simulink model "Lab2"  (R2022a)
settings: Solver=VariableStepAuto  StartTime=0.0  StopTime=100  RelTol=1e-3
values from neighbouring files (symbols this model uses):
  a = 1    [code2.m]
  am = 2    [code2.m]
  b = 0.5    [code2.m]
  bm = 2    [code2.m]
  gamma_tild = gamma*b/am    (= 5)    [code2.m]
settings Model: Creator=fades  LastModifiedBy=fades

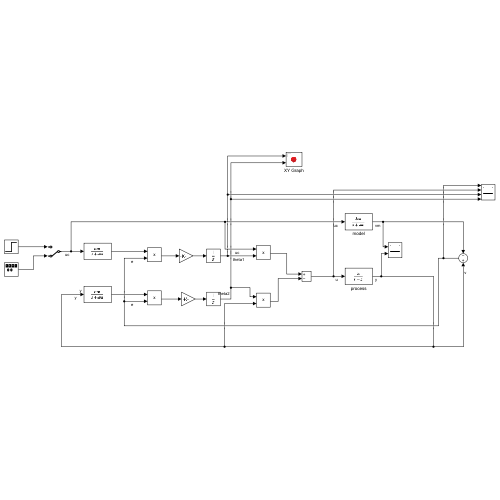
[thumbnail: Simulink's stored preview of the top-level diagram]
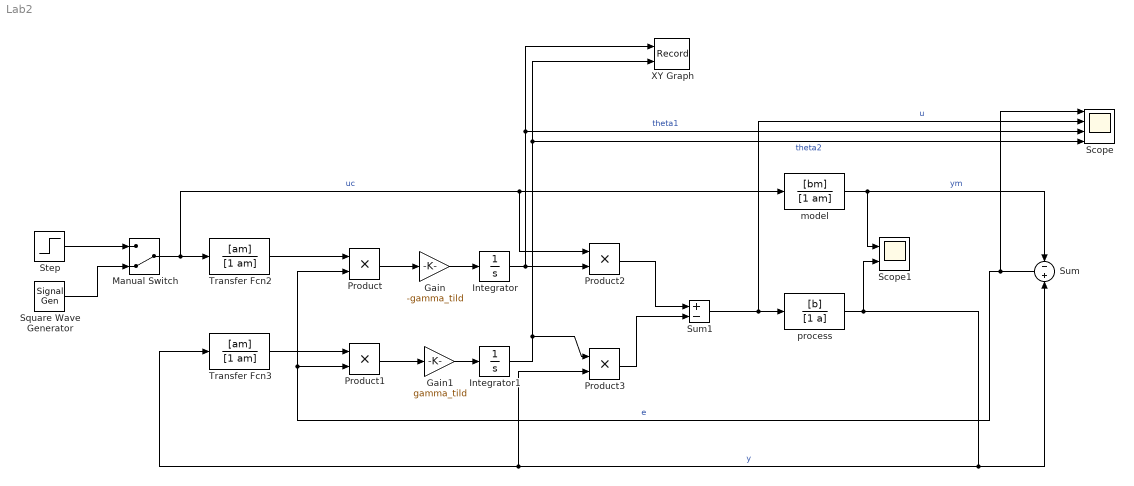
== system Lab2 ==
  Gain : Gain  Gain=-gamma_tild
  Gain1 : Gain  Gain=gamma_tild
  Integrator : Integrator
  Integrator1 : Integrator
  Manual Switch : ManualSwitch  CurrentSetting=0
  Product{,1..3} (4 alike) : Product
  Scope : Scope  NumInputPorts=4
  Scope1 : Scope  NumInputPorts=2
  Square Wave Generator : SignalGenerator  WaveForm=square  Frequency=0.05
  Step : Step  After=0.01  SampleTime=0
  Sum : Sum  Inputs=-+
  Sum1 : Sum  Inputs=+-
  Transfer Fcn2 : TransferFcn  Numerator=[am]  Denominator=[1 am]
  Transfer Fcn3 : TransferFcn  Numerator=[am]  Denominator=[1 am]
  XY Graph : Record  FileSettingsInternal="{\"entries\":[{\"content\":{\"excelSettings\":{\"content\":{},\"type\":\"Streamout.ExcelSettings\"}},\"type\":\"Streamout.FileSettingStorage\",\"uuid\":\"33b553c0-aa13-4359-a434-9299916228b1\"}],\"packageUris\":[\"http://schema.mathworks.com/mf0/streamout_blocks/R2020a\"],\"version\":\"1.0\"}"  Layout=[1 1]  SignalsInternal="{\"entries\":[{\"content\":{\"signals\":[{\"content\":{\"blockPath\":[\"Lab2/XY Graph\"],\"channel\":[],\"dimensions\":[1],\"domain\":\"Lab2/XY Graph\",\"lineColor\":\"#a2142f\",\"plots\":[1],\"port\":1,\"sid\":[\"\"],\"signalID\":54,\"signalName\":\"theta1\"},\"type\":\"RecordBlkView.Signal\",\"uuid\":\"e47f0505-aac6-4bc9-bd3a-13fd3b7bcdd4\"},{\"content\":{\"blockPath\":[\"Lab2/XY Graph\"],\"channel\":[],\"dimensions\":[1],\"domain\":\"Lab2/XY Graph\",\"lineColor\":\"#139fff\",\"plots\":[1],\"port\":2,\"sid\":[\"\"],\"signalID\":58,\"signalName\":\"theta2\"},\"type\":\"RecordBlkView.Signal\",\"uuid\":\"f4ec79ed-9af0-4ff0-8c66-8d16f2a2f4ae\"}]},\"type\":\"RecordBlkView.InputSignals\",\"uuid\":\"98caba28-9fa0-4dd7-9e9a-6578a0787a18\"}],\"packageUris\":[\"http://schema.mathworks.com/mf0/streamout_blocks/R2020a\"],\"version\":\"1.0\"}"  VisualizationBindings="{\"xyplotplugin\":{\"info\":[{\"series\":[{\"bindingParametersList\":[{\"parameter\":\"X-Axis\",\"signalID\":54,\"signalName\":\"theta1\"},{\"parameter\":\"Y-Axis\",\"signalID\":58,\"signalName\":\"theta2\"}],\"seriesID\":32204}],\"subplotID\":1}]}}"  CompatibilityTag=XY
  model : TransferFcn  Numerator=[bm]  Denominator=[1 am]
  process : TransferFcn  Numerator=[b]  Denominator=[1 a]
  wires:
  Step/1 -> Manual Switch/1
  model/1 -> Scope1/1, Sum/1  "ym"
  process/1 -> Scope1/2, Transfer Fcn3/1, Product3/2, Sum/2  "y"
  Manual Switch/1 -> model/1, Product2/1, Transfer Fcn2/1  "uc"
  Transfer Fcn2/1 -> Product/1
  Sum/1 -> Scope/1, Product/2, Product1/2  "e"
  Product/1 -> Gain/1
  Gain/1 -> Integrator/1
  Transfer Fcn3/1 -> Product1/1
  Product1/1 -> Gain1/1
  Gain1/1 -> Integrator1/1
  Integrator/1 -> XY Graph/1, Scope/3, Product2/2  "theta1"
  Integrator1/1 -> XY Graph/2, Scope/4, Product3/1  "theta2"
  Product2/1 -> Sum1/1
  Product3/1 -> Sum1/2
  Sum1/1 -> Scope/2, process/1  "u"
  Square Wave Generator/1 -> Manual Switch/2
